simulink model "plant_with_ip_to_pdf"  (R2015b)
settings: Solver=VariableStepAuto  StartTime=0.0  StopTime=10.0  RelTol=1e-3
undefined symbols (not defined in the file): Den, Iq, Ki, Kp, Num
settings Model: Creator=Morten  LastModifiedBy=Morten

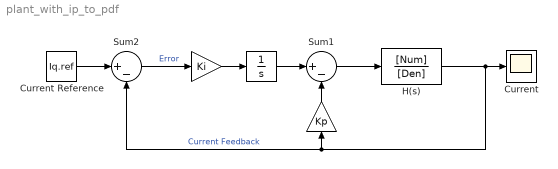
== system plant_with_ip_to_pdf ==
  " " : Integrator
  " " : Gain  Gain=Ki
  " " : Gain  Gain=Kp
  Current : Scope
  "Current Reference " : Constant  Value=Iq.ref
  H(s) : TransferFcn  Numerator=[Num]  Denominator=[Den]
  Sum1 : Sum  Inputs=|+-
  Sum2 : Sum  Inputs=|+-
  wires:
  Sum2/1 -> " "/1  "Error"
  "Current Reference "/1 -> Sum2/1
  H(s)/1 -> " "/1, Sum2/2, Current/1  "Current Feedback"
  " "/1 -> " "/1
  " "/1 -> Sum1/1
  Sum1/1 -> H(s)/1
  " "/1 -> Sum1/2
